simulink model "part_three"  (R2019b)
settings: Solver=VariableStepAuto  StartTime=0.0  StopTime=100  RelTol=1e-3
values from neighbouring files (symbols this model uses):
  delta_t = 0.001    [part_four_params.m]    (also in part_three_params.m = 0.01)
  disturbance_amplitude = -3    [part_four_params.m]    (also in part_three_params.m)
  Gs = tf(1, [1 8 13 6])    [part_four_params.m]    (also in part_three_params.m = tf([0.2], [1 2 3]))
  Kc = 1    [part_four_params.m]    (also in part_three_params.m = 10)
  step_amplitude = 10    [part_four_params.m]    (also in part_three_params.m = 3)
  target_time = 50    [part_four_params.m]    (also in part_three_params.m)
libraries: simulink x1
settings Model: Creator=adityaaaap  LastModifiedBy=adityaaaap
settings DataIOCC: ReturnWorkspaceOutputs=off
settings DebuggingCC: ArithmeticOperatorsInVariantConditions=warning
settings SFSimCC: SimUseLocalCustomCode=off  CustomCodeUndefinedFunction=UseInterfaceOnly
settings RTWCC: RTWUseLocalCustomCode=off
settings CodeAppCC: StateflowObjectComments=on

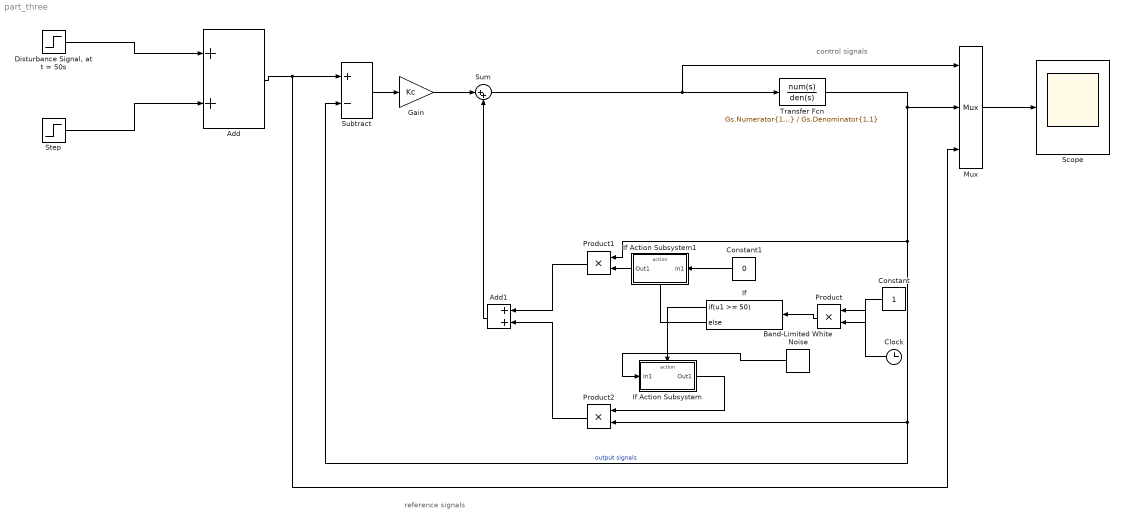
== system part_three ==
  note: control signals
  note: reference signals
  Add : Sum
  Add1 : Sum
  Band-Limited White Noise : simulink/Sources/Band-Limited White Noise  Cov=[0.1]  Ts=0.1  seed=[23341]
  Clock : Clock
  Constant : Constant
  Constant1 : Constant  Value=0
  "Disturbance Signal, at t = 50s " : Step  Time=target_time  After=disturbance_amplitude  SampleTime=0
  Gain : Gain  Gain=Kc
  If : If  IfExpression=u1 >= 50
  If Action Subsystem : Subsystem  TreatAsAtomicUnit=on
  If Action Subsystem1 : Subsystem  TreatAsAtomicUnit=on
  Mux : Mux  Inputs=3
  Product : Product
  Product1 : Product
  Product2 : Product
  Scope : Scope
  Step : Step  Time=0  After=step_amplitude  SampleTime=delta_t
  Subtract : Sum  Inputs=+-
  Sum : Sum  Inputs=|++
  Transfer Fcn : TransferFcn  Numerator=Gs.Numerator{1,1}  Denominator=Gs.Denominator{1,1}
  wires:
  Subtract/1 -> Gain/1
  Step/1 -> Add/2
  Mux/1 -> Scope/1
  Transfer Fcn/1 -> Product1/1, Product2/2, Subtract/2, Mux/2  "output signals"
  Add/1 -> Subtract/1, Mux/3
  Clock/1 -> Product/1
  Constant/1 -> Product/2
  Product/1 -> If/1
  If/1 -> If Action Subsystem/Action
  Band-Limited White Noise/1 -> If Action Subsystem/1(In1)
  If/2 -> If Action Subsystem1/Action
  Constant1/1 -> If Action Subsystem1/1(In1)
  If Action Subsystem1/1(Out1) -> Product1/2
  If Action Subsystem/1(Out1) -> Product2/1
  Product1/1 -> Add1/1
  Product2/1 -> Add1/2
  Gain/1 -> Sum/1
  Sum/1 -> Mux/1, Transfer Fcn/1
  Add1/1 -> Sum/2
  "Disturbance Signal, at t = 50s "/1 -> Add/1

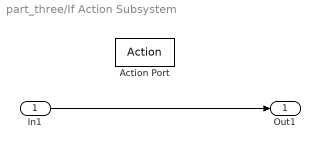
== system part_three/If Action Subsystem ==
  In1 : Inport
  Action Port : ActionPort  ActionPortLabel=if(u1 >= 50)
  Out1 : Outport
  wires:
  In1/1 -> Out1/1

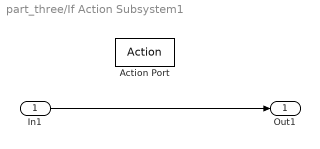
== system part_three/If Action Subsystem1 ==
  In1 : Inport
  Action Port : ActionPort  ActionPortLabel=else
  Out1 : Outport
  wires:
  In1/1 -> Out1/1
